simulink model "sampleModel195"  (R2021b)
settings: Solver=VariableStepAuto  StartTime=0.0  StopTime=10.0  RelTol=1e-3
undefined symbols (not defined in the file or in its folder): Newton, Raphson
libraries: simulink x5
settings Model: Creator=user  LastModifiedBy=user

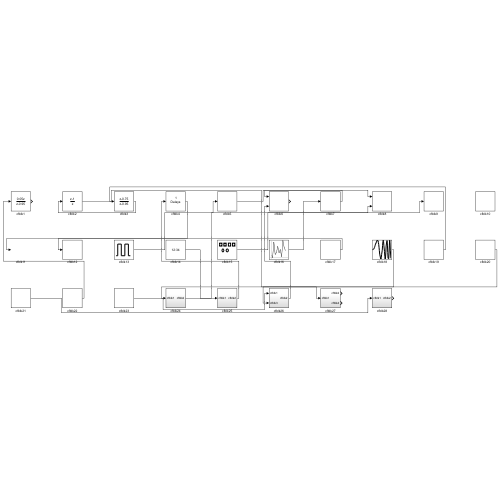
[thumbnail: Simulink's stored preview of the top-level diagram]
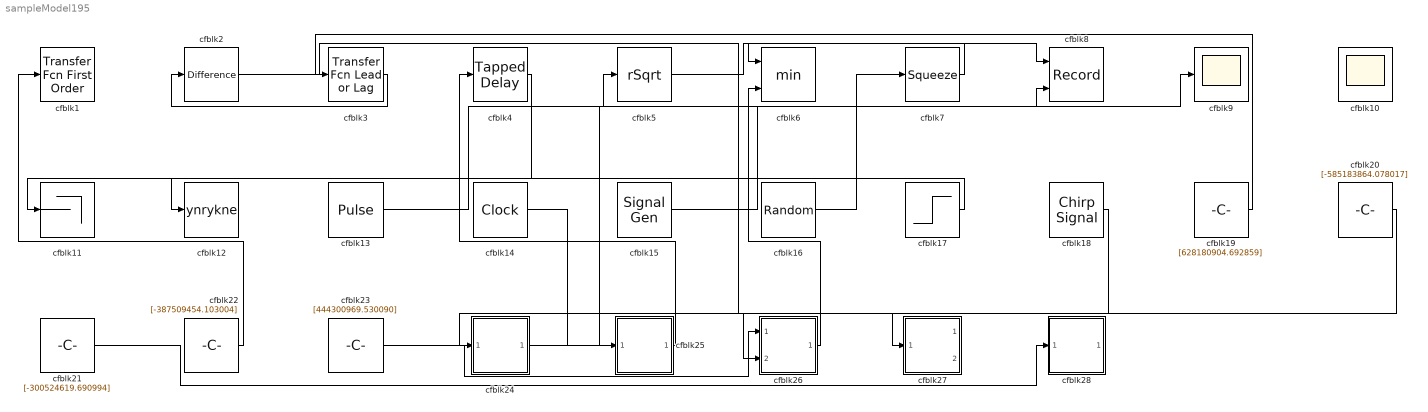
== system sampleModel195 ==
  cfblk1 : simulink/Discrete/Transfer Fcn First Order  PoleZ=0.95  ICPrevOutput=0.0  DoSatur=off
  cfblk10 : Scope
      settings: Floating=on
  cfblk11 : Terminator
  cfblk12 : ToWorkspace  VariableName=ynrykne  SaveFormat=Timeseries  SampleTime=-1
  cfblk13 : DiscretePulseGenerator  PulseType=Time based  Amplitude=[-398798093.304317]  Period=[77125726.918553]  PulseWidth=5  PhaseDelay=[4.000000]
  cfblk14 : DigitalClock
  cfblk15 : SignalGenerator  Amplitude=[-752789414.880078]
  cfblk16 : UniformRandomNumber  Minimum=[-9242255674.904612]  Maximum=[9788274661.270817]  Seed=[45810577.000000]  SampleTime=0.1
  cfblk17 : Step  Time=[5.000000]  Before=[773643221.026126]  After=[767661496.566579]  SampleTime=0
  cfblk18 : simulink/Sources/Chirp Signal  f1=[-196890405.607673]  T=[638281047.703870]  f2=[822783404.665189]
  cfblk19 : Constant  Value=[628180904.692859]  SampleTime=1
  cfblk2 : simulink/Discrete/Difference  ICPrevInput=0.0  OutMin=[]  OutMax=[]  OutDataTypeStr=Inherit: Inherit via back propagation  OutDataType=fixdt(1, 16)  OutScaling=2^-10  DoSatur=off
  cfblk20 : Constant  Value=[-585183864.078017]  SampleTime=1
  cfblk21 : Constant  Value=[-300524619.690994]  SampleTime=1
  cfblk22 : Constant  Value=[-387509454.103004]  SampleTime=1
  cfblk23 : Constant  Value=[444300969.530090]  SampleTime=1
  cfblk24 : Subsystem
  cfblk25 : Subsystem
  cfblk26 : Subsystem
  cfblk27 : Subsystem
  cfblk28 : Subsystem
  cfblk3 : simulink/Discrete/Transfer Fcn Lead or Lag  PoleZ=0.95  ZeroZ=0.75  ICPrevOutput=0.0  ICPrevInput=0.0  DoSatur=off
      settings: SourceProductBaseCode=SL
  cfblk4 : simulink/Discrete/Tapped Delay  vinit=0.0  samptime=-1  NumDelays=1  DelayOrder=Oldest  includeCurrent=off
  cfblk5 : Sqrt  Operator=rSqrt  AlgorithmType=Newton-Raphson  SaturateOnIntegerOverflow=on
  cfblk6 : MinMax  Inputs=2
  cfblk7 : Squeeze
  cfblk8 : Record  FileSettingsInternal="{\"entries\":[{\"content\":{\"excelSettings\":{\"content\":{},\"type\":\"Streamout.ExcelSettings\"}},\"type\":\"Streamout.FileSettingStorage\",\"uuid\":\"272d74a1-5d8b-46b1-9eb4-3d9c30eaade7\"}],\"packageUris\":[\"http://schema.mathworks.com/mf0/streamout_blocks/R2020a\"],\"version\":\"1.0\"}"  Layout=[1 1]  SignalsInternal="{\"entries\":[{\"content\":{\"signals\":[{\"content\":{\"blockPath\":[\"sampleModel195/cfblk8\"],\"channel\":[],\"dimensions\":[1],\"domain\":\"sampleModel195/cfblk8\",\"lineColor\":\"#a2142f\",\"plots\":[1],\"port\":1,\"sid\":[\"\"],\"signalID\":7385,\"signalName\":\"cfblk5\"},\"type\":\"RecordBlkView.Signal\",\"uuid\":\"32de41d4-8e66-4423-af7f-2e1291e0bc86\"},{\"content\":{\"blockPath\":[\"sampleModel195/cfblk8\"],\"channel\":[],\"dimensions\":[1],\"domain\":\"sampleModel195/cfblk8\",\"lineColor\":\"#139fff\",\"plots\":[1],\"port\":2,\"sid\":[\"\"],\"signalID\":7389,\"signalName\":\"cfblk15\"},\"type\":\"RecordBlkView.Signal\",\"uuid\":\"628e4f8c-79c5-4006-8f46-6c109e47f818\"}]},\"type\":\"RecordBlkView.InputSignals\",\"uuid\":\"99c10c5f-bddd-4b76-921a-7e0078a43de1\"}],\"packageUris\":[\"http://schema.mathworks.com/mf0/streamout_blocks/R2020a\"],\"version\":\"1.0\"}"  VisualizationBindings="{\"xyplotplugin\":{\"info\":[{\"series\":[{\"bindingParametersList\":[{\"parameter\":\"X-Axis\",\"signalID\":7385,\"signalName\":\"cfblk5\"},{\"parameter\":\"Y-Axis\",\"signalID\":7389,\"signalName\":\"cfblk15\"}],\"seriesID\":60012}],\"subplotID\":1}]}}"  CompatibilityTag=XY
  cfblk9 : Scope
  wires:
  cfblk14/1 -> cfblk25/1(cfblk1)
  cfblk4/1 -> cfblk11/1
  cfblk7/1 -> cfblk6/1
  cfblk22/1 -> cfblk1/1
  cfblk2/1 -> cfblk27/1(cfblk1)
  cfblk25/1(cfblk2) -> cfblk4/1
  cfblk19/1 -> cfblk3/1
  cfblk26/1(cfblk2) -> cfblk6/2
  cfblk3/1 -> cfblk2/1
  cfblk13/1 -> cfblk5/1
  cfblk23/1 -> cfblk26/1(cfblk1)
  cfblk16/1 -> cfblk7/1
  cfblk5/1 -> cfblk8/1
  cfblk17/1 -> cfblk12/1
  cfblk24/1(cfblk2) -> cfblk9/1
  cfblk20/1 -> cfblk26/2(cfblk3)
  cfblk15/1 -> cfblk8/2
  cfblk21/1 -> cfblk28/1(cfblk1)
  cfblk18/1 -> cfblk24/1(cfblk1)

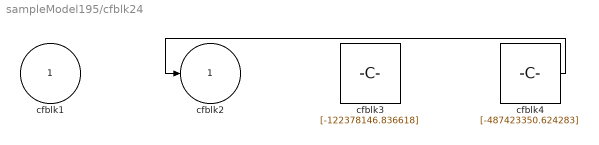
== system sampleModel195/cfblk24 ==
  cfblk1 : Inport
  cfblk3 : Constant  Value=[-122378146.836618]  SampleTime=1
  cfblk4 : Constant  Value=[-487423350.624283]  SampleTime=1
  cfblk2 : Outport
  wires:
  cfblk4/1 -> cfblk2/1

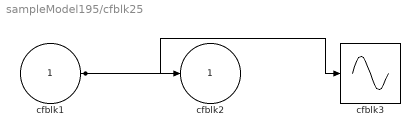
== system sampleModel195/cfblk25 ==
  cfblk1 : Inport
  cfblk3 : Sin  TimeSource=Use external signal  SampleTime=0
  cfblk2 : Outport
  wires:
  cfblk1/1 -> cfblk2/1, cfblk3/1

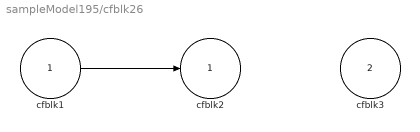
== system sampleModel195/cfblk26 ==
  cfblk1 : Inport
  cfblk3 : Inport  Port=2
  cfblk2 : Outport
  wires:
  cfblk1/1 -> cfblk2/1

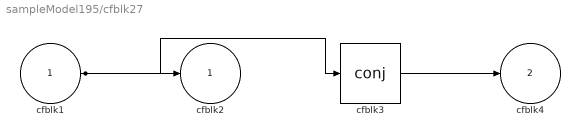
== system sampleModel195/cfblk27 ==
  cfblk1 : Inport
  cfblk3 : Math  Operator=conj  SaturateOnIntegerOverflow=on
  cfblk2 : Outport
  cfblk4 : Outport  Port=2
  wires:
  cfblk1/1 -> cfblk2/1, cfblk3/1
  cfblk3/1 -> cfblk4/1

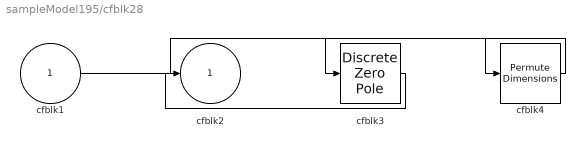
== system sampleModel195/cfblk28 ==
  cfblk1 : Inport
  cfblk3 : DiscreteZeroPole  Poles=[0 0.5]  Gain=1
  cfblk4 : PermuteDimensions
  cfblk2 : Outport
  wires:
  cfblk1/1 -> cfblk4/1
  cfblk3/1 -> cfblk2/1
  cfblk4/1 -> cfblk3/1
